simulink model "rtwdemo_udt"  (Simulink 6.0)
settings: Solver=FixedStepDiscrete  StartTime=0.0  StopTime=10  FixedStep=1  RelTol=1e-3
PostLoadFcn:
  | rtwdemo_udt_data
libraries: rtwdemowidgets x2
settings Model: Creator=The MathWorks Inc.  LastModifiedBy=batserve  ExtModeAutoUpdateStatusClock=off  ProdHWDeviceType=32-bit Embedded Processor
settings DataIOCC: SaveOutput=off  SaveTime=off  SignalLoggingName=logsOut
settings OptimizationCC: InlineParams=on  EnforceIntegerDowncast=off  StateBitsets=on  DataBitsets=on  UseTempVars=on
settings DebuggingCC: CheckExecutionContextPreStartOutputMsg=on  CheckExecutionContextRuntimeOutputMsg=on  SolverPrmCheckMsg=none
settings HardwareCC: ProdHWDeviceType=32-bit Embedded Processor  TargetHWDeviceType=32-bit Generic  ProdEqTarget=off
settings ModelReferenceCC: UpdateModelReferenceTargets=IfOutOfDate
settings RTWCC: TLCOptions=-p0 -aWarnNonSaturatedBlocks=0  GenCodeOnly=on  GenerateReport=on  RTWVerbose=off  ProcessScript=grt_make_rtw_hook  LaunchReport=on
settings CodeAppCC: ForceParamTrailComments=on

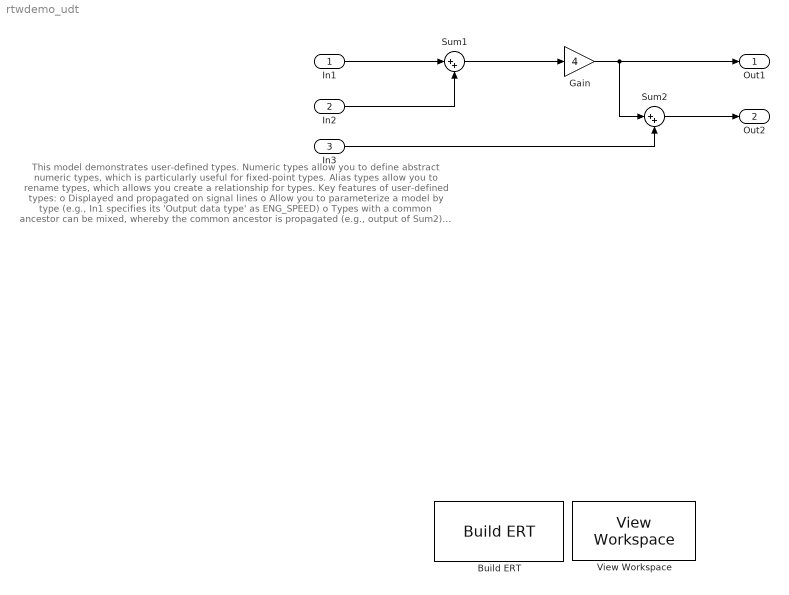
== system rtwdemo_udt ==
  note: This model demonstrates user-defined types.  Numeric types allow you to define abstract numeric types, which
      | is particularly useful for fixed-point types.  Alias types allow you to rename types, which allows you create
      | a relationship for types.  Key features of user-defined types:
      |
      | o Displayed and propagated on signal lines
      | o Allow you to parameterize a model by type (e.g., In1 specifies its 'Output data type' as ENG_SPEED)
      | o Types with a common ancestor can be mixed, whereby the common ancestor is propagated (e.g., output of Sum2)
      | o Intrinsically supported by the Simulink Model Explorer
      | o Include an optional header file attribute that is ideal for importing legacy types (ignored for GRT targets)
      | o Types used in the generated code (ignored for GRT targets)
      |
      | Try the following:
      |
      | 1) Inspect the user-defined types in the Model Explorer (View->Model Explorer), or double-click the yellow
      |     button below.  You will find ENG_SPEED and S16 in the Base Workspace node
      | 2) Compile the diagram to display the types in this model (Edit->Update Diagram)
      | 3) Generate code with the blue button below and inspect model files to see how user-defined types
      |     appear in the generated code
      | 4) Modify the attributes of ENG_SPEED and S16 and repeat steps 1-3
  In1 : Inport  Port=1  DataType=Specify via dialog  OutDataType=ENG_SPEED  LatchInput=off
  In2 : Inport  Port=2  DataType=Specify via dialog  OutDataType=ENG_SPEED  LatchInput=off
  In3 : Inport  Port=3  DataType=Specify via dialog  OutDataType=S16  LatchInput=off
  Build ERT : rtwdemowidgets/Build ERT  attrib_overrides={}
  Gain : Gain  Gain=4  OutDataTypeMode=Specify via dialog  OutDataType=ENG_SPEED
  Sum1 : Sum  Inputs=|++
  Sum2 : Sum  Inputs=|++
  View Workspace : rtwdemowidgets/View Workspace
  Out1 : Outport
  Out2 : Outport  Port=2
  wires:
  In2/1 -> Sum1/2
  In1/1 -> Sum1/1
  Sum1/1 -> Gain/1
  Gain/1 -> Out1/1, Sum2/1
  In3/1 -> Sum2/2
  Sum2/1 -> Out2/1
